simulink model "F16ASYM_Controlled_ACC"  (R2012b)
settings: Solver=ode3  SolverMode=SingleTasking  StartTime=0.0  StopTime=inf  FixedStep=T_sim  RelTol=1e-3
InitFcn:
  | load('NN_c_weights_Last_stable.mat')
values from neighbouring files (symbols this model uses):
  a1 = fitresult.p1    [Stall_protection.m]
  alpha_map_eval = ones(size(M_eval))*NaN    [Auto_trim_aid.m]    (also in Autotrim_maps.mat = [nan nan 0.277598136245 0.119432432992 0.0579479097061 0.027)
  beta_map_eval = ones(size(M_eval))*NaN    [Auto_trim_aid.m]    (also in Autotrim_maps.mat = [nan nan -0.00151549403324 0.00117807579006 -0.0052086799721)
  C_L_0 = fitresult.p2    [Stall_protection.m]
  G_eval = NaN*ones(size(M_sq,2),size(H_sq,2))    [Stall_protection.m]
  H_sq = unique(sort(H_sq))    [Stall_protection.m]
  H_sq_autotrim = min( F_envelope.H_1g):2000:max(F_envelope.H_1g)    [Auto_trim_aid.m]    (also in Autotrim_maps.mat = [0 2000 4000 6000 8000 10000 12000 14000 16000 18000])
  K_b_ACC = params(3)    [Cost_function.m]
  K_b_q = params(4)    [Cost_function.m]
  learning = 20    [Scheduling_desing.m]
  M_sq = unique(sort(M_sq))    [Stall_protection.m]
  M_sq_autotrim = 0:0.1:max(F_envelope.M_1g)    [Auto_trim_aid.m]    (also in Autotrim_maps.mat = [0 0.1 0.2 0.3 0.4 0.5 0.6 0.7 0.8 0.9 1 1.1 ... (21 element)
  Model_used_flag = 1    [Scheduling_desing.m]
  reg_param = 1    [Scheduling_desing.m]
  T_sim = 0.04    [Run_me.m]    (also in Scheduling_desing.m = 0.02)
  tau_ACC = params(1)    [Cost_function.m]
  tau_q = params(2)    [Cost_function.m]
  V_Comp_A_w_z_last = [-0.043311742939 0.0085685727899 -0.0213735657625 0.0330213821126 -0.0306555996667 -0.00573122365227 -0.0106441480787 0.0329440631876 0.0177121952361 -0.0290685435098 -0.0181457235686 -0.0361990502411 ... (1250 elements, 50x25)]    [NN_c_weights_Last_stable.mat]
  V_Comp_last = [-0.0421958473648 0.0184516098779 -0.0436695953504 -0.041154016657 0.00216882652165 -0.0388561228631 0.0327521861474 0.0326079628857 0.0227071838361 -0.0338588476214 0.0161615063846 0.00186003522421 ... (1250 elements, 50x25)]    [NN_c_weights_Last_stable.mat]
  velocity = M_eval(I,J)*a    [Auto_trim_aid.m]    (also in Scheduling_desing.m = M_eval_sche(I,J)*a)
  W_Comp_A_w_z_last = [-0.00689921461652 0.00234704735165 -0.000126421245896 0.00121944724496 6.17702028018e-05 -0.000422762754226 -0.000228913732743 -1.1618795843e-05 7.94007436465e-05 0.000588815786054 2.98617078429e-05 -0.00020420127191 ... (153 elements, 3x51)]    [NN_c_weights_Last_stable.mat]
  W_Comp_last = [-0.00864477030284 0.000183920433695 -0.000300268209456 0.00178165628538 -0.000144806488148 -0.000715209966 -0.000733452792184 5.9552378004e-05 0.000293789747621 0.00184648331608 -0.000150090451416 -0.000741280397229 ... (153 elements, 3x51)]    [NN_c_weights_Last_stable.mat]
undefined symbols (not defined in the file or in its folder): B, DiscIntNeverNeededParam, fi_flag_Simulink, k_B, m_B, sigbuilder_block, Stall_curve, Theta_1_roll_last, Theta_2_roll_last, Theta_3_roll_last, trim_control, trim_state, trim_throttle, V_long_lastA_w_z, V_long_lastAoA, V_roll_last, V_roll_lastMOD, V_yaw_last, W_long_lastA_w_z, W_long_lastAoA, W_roll_last, W_roll_lastMOD, W_yaw_last
libraries: Adaptive_FaultTolerantControl x43, F16_Actuator_Library x14, dspsigops x13, simulink x8, dsparch4 x6, simulink_extras x5, aerolibatmos2 x5, aerolibtransform2 x5, dspmtrx3 x3, qcatlib x2, dspvision x2, dspsnks4 x2
(part 10 of 10)

== matlab function F16ASYM_Controlled_ACC/Primary Controller/P controller + adaptive Isolated NN/On-line (adaptive) multi-layer NNs/Yaw Chanel/Yaw HL NN/Yaw NN ==
  data: X_bar input size=[12,1]; v_ad_comp output; e input; Ks input; B input; Long_learnign_rate input size=1; Long_reg_param input size=1; W input size=[1,31]; V input size=[30,12]; v_ad output; Z_norm_unit output; T_sim parameter; W_update output; V_update output
function [v_ad_comp,v_ad,Z_norm_unit,W_update,V_update]  = Yaw_NN(X_bar,e, Ks,B,Long_learnign_rate,Long_reg_param,W,V,T_sim)

%% Compute prelimiary parametes Ks(1)=K_b_alpha  and Ks(2) = K_b_q
P = [   1/Ks(1) , 1/(Ks(1)^2+Ks(1)*Ks(2));
     1/(Ks(1)^2+Ks(1)*Ks(2)) ,(Ks(1)^2+Ks(1)*Ks(2)+1)/(Ks(2)^2*Ks(1)+Ks(2)*Ks(1)^2) ];
zeta= e'*P*B;
s=zeros(30,1);
z=s;
%% Feedforward
z = V*X_bar;
s=sigmoid(V*X_bar);

sigma = [1 ; s ];
% v_ad = W*sigma;

sigma_grad = (sigma.*(ones(size(sigma))-sigma));

%% Compute the gradients or adaptation laws
Gamma_w= Long_learnign_rate; % W learnign rate
Gamma_v= Long_learnign_rate; %V learning rate
lambda = Long_reg_param;

V_dot=zeros(size(V));
W_dot=zeros(size(W'));

W_dot= -Gamma_w*(  (sigma - sigma_grad.*[1;z] ).*zeta  );
W_dot(2:end,1)= W_dot(2:end,1) - Gamma_w*lambda*norm(zeta)*(W(:,2:end))';

M = W'*zeta.*sigma_grad ;
V_dot= -Gamma_v*( M(2:end)*X_bar'  );
V_dot(:,2:end)= V_dot(:,2:end) - Gamma_v*lambda*norm(zeta).*V(:,2:end);


% % % Other way: Based on notes of Andrew NG
% % W_dot=zeros(size(W));
% % delta2=W'*zeta.*sigma_grad;
% % 
% % V_dot = - Gamma_v*( delta2(2:end)*X_bar');
% % V_dot(:,2:end)= V_dot(:,2:end) - Gamma_v*lambda*norm(zeta).*V(:,2:end);
% % 
% % W_dot = - Gamma_w*( zeta*sigma');
% % W_dot(:,2:end)= W_dot(:,2:end) - Gamma_w*lambda*norm(zeta)*(W(:,2:end));
% % 
% % W_dot = W_dot';


%% Adaptation
W_update = W + T_sim*W_dot';
V_update = V + T_sim*V_dot;

%% re-compute v_ad

z = V*X_bar;
s=sigmoid(V*X_bar);

sigma = [1 ; s(:,1) ];
v_ad = W*sigma;

%% Compute v_ad_comp
Z = [ V,zeros(size(V,1),size(W,2));
    zeros(size(W,1),size(V,2)),W];
    
Z_norm = norm(Z,'fro');
Z_max = 2*min(size(W,1),size(W,2) )*min( size(V,1),size(V,2) );
Z_norm_unit = Z_norm;

K_r0= 0.02;
K_r1= 0;
v_r0 = -K_r0*zeta;
v_r1 = -K_r1*(Z_norm+Z_max)*zeta;

v_ad_comp = v_ad + v_r1 +v_r0;


end

== matlab function F16ASYM_Controlled_ACC/NDI/NDI: RECONFIG/Pre-Inverter ==
  data: p_dot_comm input; L_comm output; q_dot_comm input; r_dot_comm input; M_comm output; N_comm output; omega_b input
function [L_comm,M_comm,N_comm] = Pre_inverter(p_dot_comm,q_dot_comm,r_dot_comm,omega_b)
Jy  = 75673.6;
Jxz = 1331.4; 
Jz  = 85552.1;  
Jx  = 12874.8;
h_E = 216.9;

Gamma = Jx * Jz - (Jxz  * Jxz);
C1 = ((Jy - Jz)  * Jz  - (Jxz * Jxz))/ Gamma;
C2 = ((Jx - Jy + Jz ) * Jxz ) / Gamma;
C3 = Jz / Gamma;
C4 = Jxz / Gamma;
C5 = (Jz - Jx) / Jy;
C6 = Jxz / Jy ;
C7 = 1 / Jy;
C8 = (Jx * (Jx - Jy ) + Jxz * Jxz) / Gamma;
C9 = Jx / Gamma;



L_comm = -( C4*r_dot_comm+(C2*C9-C4*C8)*omega_b(1)*omega_b(2)+(C2*C4+C1*C9)*omega_b(2)*omega_b(3)-C9*p_dot_comm )/(C3*C9-C4^2);

M_comm = (q_dot_comm-C5*omega_b(1)*omega_b(3)+C6*omega_b(1)^2-C6*omega_b(3)^2 +C7*h_E*omega_b(3))/C7;

N_comm = ( C3*r_dot_comm-C4*p_dot_comm+(C4*C1+C3*C2)*omega_b(2)*omega_b(3)+(C4*C2-C3*C8)*omega_b(1)*omega_b(2)+(C4^2-C3*C9)*h_E*omega_b(2) )/(C3*C9-C4^2);

== matlab function F16ASYM_Controlled_ACC/Primary Controller/P controller + adaptive Isolated NN/On-line (adaptive) multi-layer NNs SIMPL/Long Chanel/Long HL NN A_w_z/Long NN ==
  data: X_bar input size=[10,1]; v_ad_comp output; e input; F input; Ks input; B input; Long_learnign_rate input size=1; Long_reg_param input size=1; W input size=[1,31]; V input size=[30,10]; v_ad output; Z_norm_unit output; T_sim parameter; W_update output; V_update output
function [v_ad_comp,v_ad,Z_norm_unit,W_update,V_update]  = Long_AoA_NN(X_bar,e, F, Ks,B,Long_learnign_rate,Long_reg_param,W,V,T_sim)

%% Compute prelimiary parametes Ks(1)=K_b_alpha  and Ks(2) = K_b_q
P = [   1/Ks(1) , F/(Ks(1)^2+Ks(1)*Ks(2));
     1/(Ks(1)^2+Ks(1)*Ks(2)) ,(Ks(1)^2+Ks(1)*Ks(2)+F^2)/(Ks(2)^2*Ks(1)+Ks(2)*Ks(1)^2) ];
zeta= e'*P*B;
s=zeros(30,1);
z=s;
%% Feedforward
z = V*X_bar;
s=sigmoid(V*X_bar);

sigma = [1 ; s ];
% v_ad = W*sigma;

sigma_grad = (sigma.*(ones(size(sigma))-sigma));

%% Compute the gradients or adaptation laws
Gamma_w= Long_learnign_rate; % W learnign rate
Gamma_v= Long_learnign_rate; %V learning rate
lambda = Long_reg_param;

V_dot=zeros(size(V));
W_dot=zeros(size(W'));

W_dot= -Gamma_w*(  (sigma - sigma_grad.*[1;z] ).*zeta  );
W_dot(2:end,1)= W_dot(2:end,1) - Gamma_w*lambda*norm(zeta)*(W(:,2:end))';

M = W'*zeta.*sigma_grad ;
V_dot= -Gamma_v*( M(2:end)*X_bar'  );
V_dot(:,2:end)= V_dot(:,2:end) - Gamma_v*lambda*norm(zeta).*V(:,2:end);


% % % Other way: Based on notes of Andrew NG
% % W_dot=zeros(size(W));
% % delta2=W'*zeta.*sigma_grad;
% % 
% % V_dot = - Gamma_v*( delta2(2:end)*X_bar');
% % V_dot(:,2:end)= V_dot(:,2:end) - Gamma_v*lambda*norm(zeta).*V(:,2:end);
% % 
% % W_dot = - Gamma_w*( zeta*sigma');
% % W_dot(:,2:end)= W_dot(:,2:end) - Gamma_w*lambda*norm(zeta)*(W(:,2:end));
% % 
% % W_dot = W_dot';


%% Adaptation
W_update = W + T_sim*W_dot';
V_update = V + T_sim*V_dot;

%% re-compute v_ad

z = V*X_bar;
s=sigmoid(V*X_bar);

sigma = [1 ; s(:,1) ];
v_ad = W*sigma;

%% Compute v_ad_comp
Z = [ V,zeros(size(V,1),size(W,2));
    zeros(size(W,1),size(V,2)),W];
    
Z_norm = norm(Z,'fro');
Z_max = 2*min(size(W,1),size(W,2) )*min( size(V,1),size(V,2) );
Z_norm_unit = Z_norm/Z_max;

K_r0= 0.1;
K_r1= 0.001;
v_r0 = -K_r0*zeta;
v_r1 = -K_r1*(Z_norm+Z_max)*zeta;

v_ad_comp = v_ad + v_r1 +v_r0;


end

== matlab function F16ASYM_Controlled_ACC/Primary Controller/P controller + adaptive Isolated NN/On-line (adaptive) multi-layer NNs SIMPL/Long Chanel/Long HL NN AoA/Long NN ==
  data: X_bar input size=[10,1]; v_ad_comp output; e input; Ks input; B input; Long_learnign_rate input size=1; Long_reg_param input size=1; W input size=[1,31]; V input size=[30,10]; v_ad output; Z_norm_unit output; T_sim parameter; W_update output; V_update output
function [v_ad_comp,v_ad,Z_norm_unit,W_update,V_update]  = Long_AoA_NN(X_bar,e, Ks,B,Long_learnign_rate,Long_reg_param,W,V,T_sim)

%% Compute prelimiary parametes Ks(1)=K_b_alpha  and Ks(2) = K_b_q
P = [   1/Ks(1) , 1/(Ks(1)^2+Ks(1)*Ks(2));
     1/(Ks(1)^2+Ks(1)*Ks(2)) ,(Ks(1)^2+Ks(1)*Ks(2)+1)/(Ks(2)^2*Ks(1)+Ks(2)*Ks(1)^2) ];
zeta= e'*P*B;
s=zeros(30,1);
z=s;
%% Feedforward
z = V*X_bar;
s=sigmoid(V*X_bar);

sigma = [1 ; s ];
% v_ad = W*sigma;

sigma_grad = (sigma.*(ones(size(sigma))-sigma));

%% Compute the gradients or adaptation laws
Gamma_w= Long_learnign_rate; % W learnign rate
Gamma_v= Long_learnign_rate; %V learning rate
lambda = Long_reg_param;

V_dot=zeros(size(V));
W_dot=zeros(size(W'));

W_dot= -Gamma_w*(  (sigma - sigma_grad.*[1;z] ).*zeta  );
W_dot(2:end,1)= W_dot(2:end,1) - Gamma_w*lambda*norm(zeta)*(W(:,2:end))';

M = W'*zeta.*sigma_grad ;
V_dot= -Gamma_v*( M(2:end)*X_bar'  );
V_dot(:,2:end)= V_dot(:,2:end) - Gamma_v*lambda*norm(zeta).*V(:,2:end);


% % % Other way: Based on notes of Andrew NG
% % W_dot=zeros(size(W));
% % delta2=W'*zeta.*sigma_grad;
% % 
% % V_dot = - Gamma_v*( delta2(2:end)*X_bar');
% % V_dot(:,2:end)= V_dot(:,2:end) - Gamma_v*lambda*norm(zeta).*V(:,2:end);
% % 
% % W_dot = - Gamma_w*( zeta*sigma');
% % W_dot(:,2:end)= W_dot(:,2:end) - Gamma_w*lambda*norm(zeta)*(W(:,2:end));
% % 
% % W_dot = W_dot';


%% Adaptation
W_update = W + T_sim*W_dot';
V_update = V + T_sim*V_dot;

%% re-compute v_ad

z = V*X_bar;
s=sigmoid(V*X_bar);

sigma = [1 ; s(:,1) ];
v_ad = W*sigma;

%% Compute v_ad_comp
Z = [ V,zeros(size(V,1),size(W,2));
    zeros(size(W,1),size(V,2)),W];
    
Z_norm = norm(Z,'fro');
Z_max = 2*min(size(W,1),size(W,2) )*min( size(V,1),size(V,2) );
Z_norm_unit = Z_norm;

K_r0= 0.02;
K_r1= 0;
v_r0 = -K_r0*zeta;
v_r1 = -K_r1*(Z_norm+Z_max)*zeta;

v_ad_comp = v_ad + v_r1 +v_r0;


end

== matlab function F16ASYM_Controlled_ACC/Primary Controller/P controller + adaptive Isolated NN/On-line (adaptive) multi-layer NNs SIMPL/Yaw Chanel/Yaw HL NN/Yaw NN ==
  data: X_bar input size=[12,1]; v_ad_comp output; e input; Ks input; B input; Long_learnign_rate input size=1; Long_reg_param input size=1; W input size=[1,31]; V input size=[30,12]; v_ad output; Z_norm_unit output; T_sim parameter; W_update output; V_update output
function [v_ad_comp,v_ad,Z_norm_unit,W_update,V_update]  = Yaw_NN(X_bar,e, Ks,B,Long_learnign_rate,Long_reg_param,W,V,T_sim)

%% Compute prelimiary parametes Ks(1)=K_b_alpha  and Ks(2) = K_b_q
P = [   1/Ks(1) , 1/(Ks(1)^2+Ks(1)*Ks(2));
     1/(Ks(1)^2+Ks(1)*Ks(2)) ,(Ks(1)^2+Ks(1)*Ks(2)+1)/(Ks(2)^2*Ks(1)+Ks(2)*Ks(1)^2) ];
zeta= e'*P*B;
s=zeros(30,1);
z=s;
%% Feedforward
z = V*X_bar;
s=sigmoid(V*X_bar);

sigma = [1 ; s ];
% v_ad = W*sigma;

sigma_grad = (sigma.*(ones(size(sigma))-sigma));

%% Compute the gradients or adaptation laws
Gamma_w= Long_learnign_rate; % W learnign rate
Gamma_v= Long_learnign_rate; %V learning rate
lambda = Long_reg_param;

V_dot=zeros(size(V));
W_dot=zeros(size(W'));

W_dot= -Gamma_w*(  (sigma - sigma_grad.*[1;z] ).*zeta  );
W_dot(2:end,1)= W_dot(2:end,1) - Gamma_w*lambda*norm(zeta)*(W(:,2:end))';

M = W'*zeta.*sigma_grad ;
V_dot= -Gamma_v*( M(2:end)*X_bar'  );
V_dot(:,2:end)= V_dot(:,2:end) - Gamma_v*lambda*norm(zeta).*V(:,2:end);


% % % Other way: Based on notes of Andrew NG
% % W_dot=zeros(size(W));
% % delta2=W'*zeta.*sigma_grad;
% % 
% % V_dot = - Gamma_v*( delta2(2:end)*X_bar');
% % V_dot(:,2:end)= V_dot(:,2:end) - Gamma_v*lambda*norm(zeta).*V(:,2:end);
% % 
% % W_dot = - Gamma_w*( zeta*sigma');
% % W_dot(:,2:end)= W_dot(:,2:end) - Gamma_w*lambda*norm(zeta)*(W(:,2:end));
% % 
% % W_dot = W_dot';


%% Adaptation
W_update = W + T_sim*W_dot';
V_update = V + T_sim*V_dot;

%% re-compute v_ad

z = V*X_bar;
s=sigmoid(V*X_bar);

sigma = [1 ; s(:,1) ];
v_ad = W*sigma;

%% Compute v_ad_comp
Z = [ V,zeros(size(V,1),size(W,2));
    zeros(size(W,1),size(V,2)),W];
    
Z_norm = norm(Z,'fro');
Z_max = 2*min(size(W,1),size(W,2) )*min( size(V,1),size(V,2) );
Z_norm_unit = Z_norm;

K_r0= 0.02;
K_r1= 0;
v_r0 = -K_r0*zeta;
v_r1 = -K_r1*(Z_norm+Z_max)*zeta;

v_ad_comp = v_ad + v_r1 +v_r0;


end

== matlab function F16ASYM_Controlled_ACC/Primary Controller/P controller + adaptive Crossed NN + AWU+Lim /Physical limitation/max deflections estimator ==
  data: v_comm input; max_defl output; B parameter
function max_defl = Max_defl(v_comm,B)
sup_limit = [24,24,21,21,29,25,25];
inf_limit = [-24,-24,-21,-21,-29,0,0];

def=B;
for i=1:3
    def(i,:) = B(i,:).*sign(v_comm(i));
end
def_avg = mean(def,1);

max_defl = zeros(7,1);
for i=1:7
    if def_avg(1,i)>0
        max_defl(i) = sup_limit(i);
    else
        max_defl(i) = inf_limit(i);
    end
end

== matlab function F16ASYM_Controlled_ACC/Anti-windup Calculation/Anti-windup: NO reconfigurable/Ang Accel ==
  data: L input; p_dot output; q_dot output; r_dot output; M input; N input; omega_b input
function [p_dot,q_dot,r_dot] = Ang_accel(L,M,N,omega_b)
Jy  = 75673.6;
Jxz = 1331.4; 
Jz  = 85552.1;  
Jx  = 12874.8;
h_E = 216.9;

denom = Jx*Jz - Jxz*Jxz;

% % C1 = ((Jy - Jz)  * Jz  - (Jxz * Jxz))/ Gamma;
% % C2 = ((Jx - Jy + Jz ) * Jxz ) / Gamma;
% % C3 = Jz / Gamma;
% % C4 = Jxz / Gamma;
% % C5 = (Jz - Jx) / Jy;
% % C6 = Jxz / Jy ;
% % C7 = 1 / Jy;
% % C8 = (Jx * (Jx - Jy ) + Jxz * Jxz) / Gamma;
% % C9 = Jx / Gamma;


p_dot =  (Jz*L + Jxz*N - (Jz*(Jz-Jy)+Jxz*Jxz)*omega_b(2)*omega_b(3) + Jxz*(Jx-Jy+Jz)*omega_b(1)*omega_b(2) + Jxz*omega_b(2)*h_E)/denom;

q_dot = (M + (Jz-Jx)*omega_b(1)*omega_b(3) - Jxz*(omega_b(1)*omega_b(1)-omega_b(3)*omega_b(3)) - omega_b(3)*h_E)/Jy;


r_dot = (Jx*N + Jxz*L + (Jx*(Jx-Jy)+Jxz*Jxz)*omega_b(1)*omega_b(2) - Jxz*(Jx-Jy+Jz)*omega_b(2)*omega_b(3) +  Jx*omega_b(2)*h_E)/denom;

== matlab function F16ASYM_Controlled_ACC/Primary Controller/P controller + adaptive Crossed NN + AWU+Lim /Complete crossed On-line (adaptive) multi-layer NN/Complete crossed On-line (adaptive) multi-layer NN: A_w_z/Cross NN A_w_z ==
  data: X_bar input size=[25,1]; v_ad_comp output; e input; Factor_F input; K_roll input; Ks_long input; Ks_yaw input; B input; Learnign_rate input size=1; Reg_param input size=1; AWU input; W input size=[3,51]; V input size=[50,25]; v_ad output; Z_norm_unit output; T_sim parameter; W_update output; V_update output
function [v_ad_comp,v_ad,Z_norm_unit,W_update,V_update]  = Cross_NN(X_bar,e,Factor_F, K_roll,Ks_long,Ks_yaw,B,Learnign_rate,Reg_param,AWU,W,V,T_sim)

%% Compute prelimiary parametes
% Compute P with regular Lyapunov equation solution
P_roll=1/K_roll;
P_long =  [   1/Ks_long(1) , Factor_F/(Ks_long(1)^2+Ks_long(1)*Ks_long(2));
     1/(Ks_long(1)^2+Ks_long(1)*Ks_long(2)) ,(Ks_long(1)^2+Ks_long(1)*Ks_long(2)+Factor_F^2)/(Ks_long(2)^2*Ks_long(1)+Ks_long(2)*Ks_long(1)^2) ];
P_yaw = [   1/Ks_yaw(1) , 1/(Ks_yaw(1)^2+Ks_yaw(1)*Ks_yaw(2));
     1/(Ks_yaw(1)^2+Ks_yaw(1)*Ks_yaw(2)) ,(Ks_yaw(1)^2+Ks_yaw(1)*Ks_yaw(2)+1)/(Ks_yaw(2)^2*Ks_yaw(1)+Ks_yaw(2)*Ks_yaw(1)^2) ];
 
P = blkdiag(P_roll,P_long,P_yaw);

% % % % Compute P with on-line Lyapunov equation solution
% % % CROSS = 0;
% % % A = [ -K_roll,0,CROSS,0,0;0,-Ks_long(1),1,0,0;
% % %     0,0,-Ks_long(2),0,0;0,0,0,-Ks_yaw(1),Factor_F;0,0,0,0,-Ks_yaw(2)];
% % % 
% % % coder.extrinsic('lyap')
% % % P = A;
% % % P = lyap(A,2*diag(ones(5,1)));



K_awu = 1.2;
zeta= e'*P*B;


% Introduce Anti-windup
zeta = zeta - K_awu*AWU'.*T_sim; 

% Convergence limitation
if norm(zeta)>2/(T_sim*Learnign_rate*Reg_param)
    zeta = (zeta./norm(zeta)).*(1.8/(T_sim*Learnign_rate*Reg_param));
end

%% Feedforward
z = V*X_bar;
s=sigmoid(V*X_bar);

sigma = [1 ; s ];
% v_ad = W*sigma;

sigma_grad = (sigma.*(ones(size(sigma))-sigma));

%% Compute the gradients or adaptation laws
Gamma_w= Learnign_rate; % W learnign rate
Gamma_v= Learnign_rate; %V learning rate
lambda = Reg_param;

V_dot=zeros(size(V));
W_dot=zeros(size(W));

W_dot= -Gamma_w*(  (sigma - sigma_grad.*[1;z] )*zeta  )';
W_dot(:,2:end)= W_dot(:,2:end) - Gamma_w*lambda*norm(zeta)*(W(:,2:end));

M = W'*zeta'.*sigma_grad ;
V_dot= -Gamma_v*( M(2:end)*X_bar'  );
V_dot(:,2:end)= V_dot(:,2:end) - Gamma_v*lambda*norm(zeta).*V(:,2:end);

% % % Other way: Based on notes of Andrew NG
% % 
% % delta2=W'*zeta'.*sigma_grad;
% % 
% % V_dot = - Gamma_v*( delta2(2:end)*X_bar');
% % V_dot(:,2:end)= V_dot(:,2:end) - Gamma_v*lambda*norm(zeta).*V(:,2:end);
% % 
% % W_dot = - Gamma_w*( sigma*zeta)';
% % W_dot(:,2:end)= W_dot(:,2:end) - Gamma_w*lambda*norm(zeta)*(W(:,2:end));



%% Adaptation
W_update = W + T_sim*W_dot;
V_update = V + T_sim*V_dot;
% 
%% Re-compute v_ad

s=sigmoid(V_update*X_bar);

sigma = [1 ; s(:,1) ];
v_ad = W_update*sigma;

%% Compute v_ad_comp
Z = [ V,zeros(size(V,1),size(W,2));
    zeros(size(W,1),size(V,2)),W];
    
Z_norm = norm(Z,'fro');
Z_max = 2*min(size(W,1),size(W,2) )*min( size(V,1),size(V,2) );
Z_norm_unit = Z_norm;

K_r0= 0;
K_r1= 0;
v_r0 = -K_r0*zeta';
v_r1 = -K_r1*(Z_norm+Z_max)*zeta';

v_ad_comp = v_ad + v_r1 +v_r0;

% % % Normalization of matrices
% % if Z_norm>Z_max
% %     V = (V.*Z_max)./Z_norm;
% %     W = (W.*Z_max)./Z_norm;
% % end
end
